simulink model "Mealy"  (R2020a)
settings: Solver=VariableStepAuto  StartTime=0.0  StopTime=5  RelTol=1e-3
settings Model: Creator=none  LastModifiedBy=none

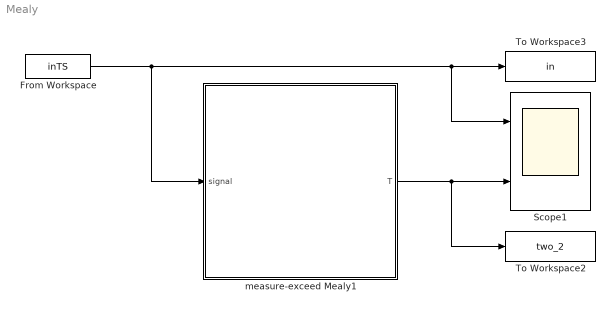
== system Mealy ==
  From Workspace : FromWorkspace  VariableName=inTS  SampleTime=1
  Scope1 : Scope  NumInputPorts=2
  To Workspace2 : ToWorkspace  VariableName=two_2  SaveFormat=Timeseries  SampleTime=-1
  To Workspace3 : ToWorkspace  VariableName=in  SaveFormat=Timeseries  SampleTime=-1
  measure-exceed Mealy1 : Stateflow chart  TreatAsAtomicUnit=on
  wires:
  measure-exceed Mealy1/1(T) -> To Workspace2/1, Scope1/2
  From Workspace/1 -> measure-exceed Mealy1/1(signal), Scope1/1, To Workspace3/1

== stateflow chart Mealy/measure-exceed Mealy1 ==
  settings: stateMachineType=MEALY_MACHINE  initializeOutput=1
  state checking for unsure [group]
    state a5
    state a4
    state a6
    state a
    state a13
    state a14
    state a12
    state a1
    state a3
    a5 -> a5 [order 2] : [signal==1&&one~=5&&cnt!=7]{cnt=cnt+1,one=one+1,T=1}
    a4 -> a5 [order 2] : [signal==1&&cnt!=7]{cnt=cnt+1,one=one+1,T=1}
    a14 -> a5 [order 1] : [signal==1&&cnt!=7]{cnt=cnt+1,one=one+1,T=1}
    a -> a4 [order 2] : [signal==1&&cnt!=7]{cnt=cnt+1,one=one+1,T=0}
    a4 -> a6 [order 1] : [signal==0&&cnt!=7]{cnt=cnt+1,T=1}
    a6 -> a6 [order 2] : [signal==1&&one!=5&&cnt!=7]{cnt=cnt+1,one=one+1,T=1}
    a14 -> a6 [order 3] : [signal==0&&cnt!=7]{cnt=cnt+1,T=1}
    a -> a1 [order 1] : [signal==0&&cnt!=7]{cnt=cnt+1,T=0}
    a12 -> a13 [order 1] : [signal==1&&cnt!=7]{cnt=cnt+1,one=one+1,T=0}
    a13 -> a14 [order 1] : [signal==1&&cnt!=7]{cnt=cnt+1,one=one+1,T=1}
    a13 -> a1 [order 3] : [signal==0&&cnt!=7]{cnt=cnt+1,one=one+1,T=0}
    a3 -> a3 [order 1] : [signal==1&&cnt!=7]{cnt=cnt+1,one=one+1,T=1}
    a1 -> a3 [order 2] : [signal==1&&cnt!=7]{cnt=cnt+1,one=one+1,T=1}
    a1 -> a12 [order 1] : [signal==0&&cnt!=7]{cnt=cnt+1,T=0}
    a12 -> a12 [order 2] : [signal==0&&cnt!=7]{cnt=cnt+1,T=0}
  state sure [group]
    state a19
    state a20
    state a21
    a19 -> a19 [order 1] : [signal==1&&cnt!=7]{cnt=cnt+1,one=one+1,T=2}
    a19 -> a19 [order 2] : [signal==0&&cnt!=7]{cnt=cnt+1,T=2}
    a20 -> a20 [order 1] : [signal==1&&cnt!=7]{cnt=cnt+1,one=one+1,T=2}
    a20 -> a20 [order 2] : [signal==0&&cnt!=7]{cnt=cnt+1,T=2}
    a21 -> a21 [order 1] : [signal==1&&cnt!=7]{cnt=cnt+1,one=one+1,T=2}
    a21 -> a21 [order 2] : [signal==0&&cnt!=7]{cnt=cnt+1,T=2}
  state unsure and not going to be sure [group]
    state a16
    state a17
    state a18
    a16 -> a16 [order 1] : [signal==1&&cnt!=7]{cnt=cnt+1,one=one+1,T=1}
    a16 -> a16 [order 2] : [signal==0&&cnt!=7]{cnt=cnt+1,T=1}
    a17 -> a17 [order 1] : [signal==1&&cnt!=7]{cnt=cnt+1,one=one+1,T=1}
    a17 -> a17 [order 2] : [signal==0&&cnt!=7]{cnt=cnt+1,T=1}
    a18 -> a18 [order 1] : [signal==1&&cnt!=7]{cnt=cnt+1,one=one+1,T=1}
    a18 -> a18 [order 2] : [signal==0&&cnt!=7]{cnt=cnt+1,T=1}
  state Begin
  a21 -> Begin [order 3] : [(signal==1||signal==0)&&cnt==7]{cnt=0,one=0,T=2}
  a20 -> Begin [order 3] : [(signal==1||signal==0)&&cnt==7]{cnt=0,one=0,T=2}
  a19 -> Begin [order 3] : [(signal==1||signal==0)&&cnt==7]{cnt=0,one=0,T=2}
  a6 -> Begin [order 4] : [(signal==1||signal==0)&&cnt==7]{cnt=0,one=0,T=1}
  a5 -> Begin [order 4] : [(signal==1||signal==0)&&cnt==7]{cnt=0,one=0,T=1}
  a5 -> a19 [order 3] : [signal==1&&one==5&&cnt~=7]{cnt=cnt+1,one=one+1,T=2}
  a5 -> a16 [order 1] : [signal==0&&cnt!=7]{cnt=cnt+1,T=1}
  a4 -> Begin [order 3] : [(signal==1||signal==0)&&cnt==7]{cnt=0,one=0,T=0}
  a16 -> Begin [order 3] : [(signal==1||signal==0)&&cnt==7]{cnt=0,one=0,T=1}
  a14 -> Begin [order 2] : [(signal==1||signal==0)&&cnt==7]{cnt=0,one=0,T=0}
  a13 -> Begin [order 2] : [(signal==1||signal==0)&&cnt==7]{cnt=0,one=0,T=0}
  a6 -> a20 [order 3] : [signal==1&&one==5&&cnt!=7]{cnt=cnt+1,one=one+1,T=2}
  a6 -> a17 [order 1] : [signal==0&&cnt!=7]{cnt=cnt+1,T=1}
  Begin -> a [order 1] : [signal==1]{cnt=1,one=one+1,T=0}
  (default) -> Begin : {cnt=0,one=0,T=0}
  Begin -> a12 [order 2] : [signal==0]{cnt=1,T=0}
  a1 -> Begin [order 3] : [(signal==1||signal==0)&&cnt==7]{cnt=0,one=0,T=0}
  a12 -> Begin [order 3] : [(signal==1||signal==0)&&cnt==7]{cnt=0,one=0,T=0}
  a17 -> Begin [order 3] : [(signal==1||signal==0)&&cnt==7]{cnt=0,one=0,T=1}
  a18 -> Begin [order 3] : [(signal==1||signal==0)&&cnt==7]{cnt=0,one=0,T=1}
  a3 -> Begin [order 4] : [(signal==1||signal==0)&&cnt==7]{cnt=0,one=0,T=1}
  a3 -> a21 [order 2] : [signal==1&&one==5&&cnt!=7]{cnt=cnt+1,one=one+1,T=2}
  a3 -> a18 [order 3] : [signal==0&&cnt!=7]{cnt=cnt+1,T=1}
  data: signal input; T output double; cnt local double; one local double
